simulink model "autopilot"  (R2019a)
settings: Solver=VariableStepAuto  StartTime=0.0  StopTime=250  RelTol=1e-3
values from neighbouring files (symbols this model uses):
  a_phi_1 = 2.87    [Problem_2.m]
  a_phi_2 = -0.65    [Problem_2.m]
  chi_c = deg2rad(10)    [Problem_2.m]
  d = deg2rad(1.5)    [Problem_2.m]
  g = 9.81    [Problem_2.m]
  k_d_phi = 1.9351    [Problem_2.m]
  k_i_chi = (w_n_chi^2*V_g)/g    (= 0.21351016627)    [Problem_2.m]
  k_p_chi = (2*zeta_chi*w_n_chi*V_g)/g    (= 3.74513534942)    [Problem_2.m]
  k_p_phi = -2    [Problem_2.m]
  V_g = 580/3.6    (= 161.111111111)    [Problem_2.m]
settings Model: Creator=joaki  LastModifiedBy=magnusknaedal

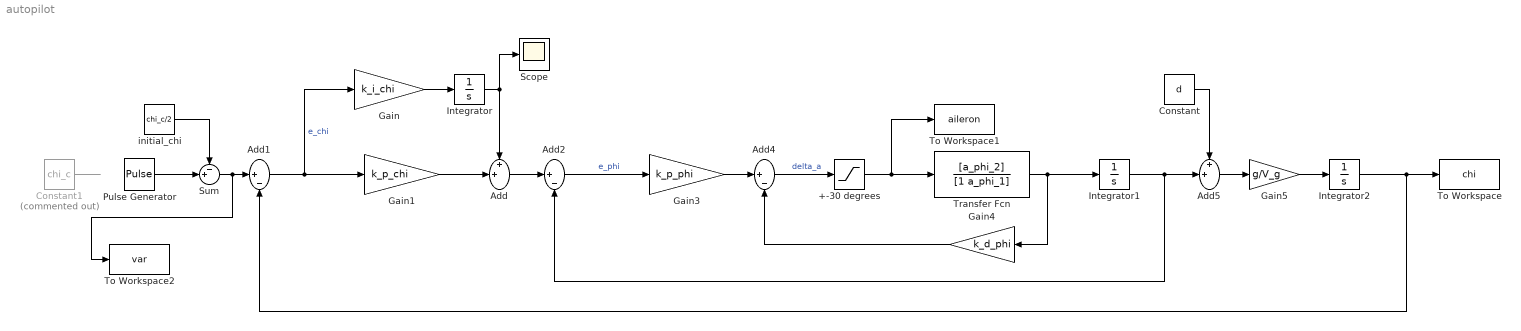
== system autopilot ==
  +-30 degrees : Saturate  UpperLimit=30*pi/180  LowerLimit=-30*pi/180
  Add : Sum  Inputs=++|
  Add1 : Sum  Inputs=|+-
  Add2 : Sum  Inputs=|+-
  Add4 : Sum  Inputs=|+-
  Add5 : Sum  Inputs=++|
  Constant : Constant  Value=d
  Constant1 : Constant  Commented=on  Value=chi_c
  Gain : Gain  Gain=k_i_chi
  Gain1 : Gain  Gain=k_p_chi
  Gain3 : Gain  Gain=k_p_phi
  Gain4 : Gain  Gain=k_d_phi
  Gain5 : Gain  Gain=g/V_g
  Integrator : Integrator
  Integrator1 : Integrator
  Integrator2 : Integrator
  Pulse Generator : DiscretePulseGenerator  PulseType=Time based  Amplitude=chi_c  Period=200  PulseWidth=50
  Scope : Scope
  Sum : Sum  Inputs=-+|
  To Workspace : ToWorkspace  VariableName=chi  SaveFormat=Timeseries  SampleTime=-1
  To Workspace1 : ToWorkspace  VariableName=aileron  SaveFormat=Timeseries  SampleTime=-1
  To Workspace2 : ToWorkspace  VariableName=var  SaveFormat=Structure With Time  SampleTime=-1
  Transfer Fcn : TransferFcn  Numerator=[a_phi_2]  Denominator=[1 a_phi_1]
  "initial_chi " : Constant  Value=chi_c/2
  wires:
  Gain/1 -> Integrator/1
  Integrator/1 -> Add/1, Scope/1
  Gain1/1 -> Add/2
  Add1/1 -> Gain/1, Gain1/1  "e_chi"
  Add2/1 -> Gain3/1  "e_phi"
  Add/1 -> Add2/1
  Gain3/1 -> Add4/1
  Transfer Fcn/1 -> Gain4/1, Integrator1/1
  Gain4/1 -> Add4/2
  Integrator1/1 -> Add5/2, Add2/2
  Constant/1 -> Add5/1
  Add5/1 -> Gain5/1
  Gain5/1 -> Integrator2/1
  Integrator2/1 -> Add1/2, To Workspace/1
  +-30 degrees/1 -> Transfer Fcn/1, To Workspace1/1
  Add4/1 -> +-30 degrees/1  "delta_a"
  "initial_chi "/1 -> Sum/1
  Constant1/1 -> ?
  Sum/1 -> To Workspace2/1, Add1/1
  Pulse Generator/1 -> Sum/2
